simulink model "RPI_fuzzy"  (R2023b)
settings: Solver=ode3  StartTime=0.0  StopTime=inf  FixedStep=1  RelTol=1e-3  EnableMultiTasking=on
InitFcn:
  | rules_fuzzy_e_de=readfis('rules_fuzzy_e_de.fis');
values from neighbouring files (symbols this model uses):
  temp_ref = 22    [RPI_Fuzzy_script.m]    (also in plot_fuzzy.m = simout(:,1))
libraries: raspberrypiIOTlib x4, raspberrypiBasiclib x2, raspberrypienvironmentalsensorslib x1, fuzblock x1
settings Model: SimulationMode=external  ExtModeTrigDuration=2  Creator=marci  LastModifiedBy=marci
settings SolverCC: PositivePriorityOrder=on  AutoInsertRateTranBlk=on
settings OptimizationCC: EnhancedBackFolding=on  PassReuseOutputArgsAs=Individual arguments  ZeroExternalMemoryAtStartup=off  ZeroInternalMemoryAtStartup=off  MaxStackSize=64  OptimizeBlockOrder=speed  DifferentSizesBufferReuse=on  OptimizationCustomize=off  EfficientTunableParamExpr=on
settings DebuggingCC: ParameterTunabilityLossMsg=error
settings HardwareCC: ProdBitPerPointer=32  ProdBitPerSizeT=32  ProdBitPerPtrDiffT=32  ProdLargestAtomicInteger=Long  ProdLargestAtomicFloat=Double  ProdWordSize=32  ProdLongLongMode=on  ProdHWDeviceType=ARM Compatible->ARM Cortex
settings RTWCC: Description=Embedded Coder  SystemTargetFile=ert.tlc  HardwareBoard=Raspberry Pi  TemplateMakefile=ert_default_tmf  Toolchain=GNU GCC Embedded Linux  BuildConfiguration=Faster Runs
settings CodeAppCC: ForceParamTrailComments=on  IgnoreCustomStorageClasses=off  OperatorAnnotations=on  SimulinkDataObjDesc=on  SFDataObjDesc=on  InsertBlockDesc=on
settings ERTTargetCC: TargetLangStandard=C99 (ISO)  SupportContinuousTime=on  SupportVariableSizeSignals=on  ExtMode=on  ExtModeTransport=2  ExtModeStaticAlloc=on  ExtModeMaxTrigDuration=1000  ExtModeMexFile=ext_xcp  ExtModeMexArgs='192.168.0.236' 0 17725  ExtModeIntrfLevel=Level2 - Open

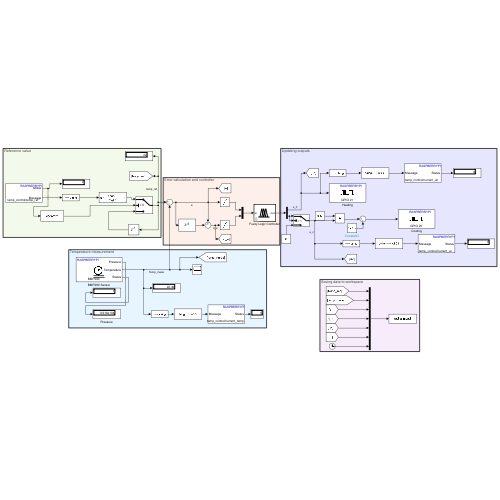
[thumbnail: Simulink's stored preview of the top-level diagram]
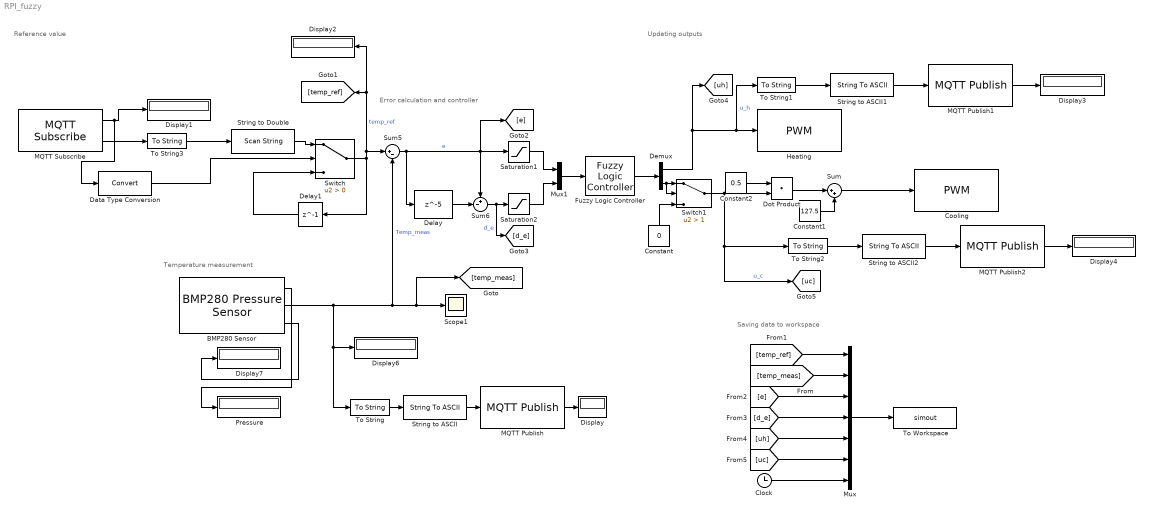
== system RPI_fuzzy ==
  note: Error calculation and controller
  note: Reference value
  note: Temperature measurement
  note: Saving data to workspace
  note: Updating outputs
  BMP280 Sensor : raspberrypienvironmentalsensorslib/BMP280 Pressure Sensor  I2CModule=1  I2CAddress=0x76  BitRate=1000000  IsActivePressure=on  IsActiveTemperature=on  IsStatus=on  FilterMode=0  PressureSensitivityFactor=2.62  TemperatureSensitivityFactor=0.005  DataType=double  SampleTime=1
  Clock : Clock
  Constant : Constant  Value=0
  Constant1 : Constant  Value=127.5
  Constant2 : Constant  Value=0.5
  Cooling : raspberrypiBasiclib/PWM  board=Pi 3 Model B  Pin_=20  Frequency=40  blockPlatform=Raspberry Pi
  Data Type Conversion : DataTypeConversion  SaturateOnIntegerOverflow=off  RndMeth=Floor
  Delay : Delay  DelayLength=5  InputProcessing=Columns as channels (frame based)  SampleTime=1
  Delay1 : Delay  DelayLength=1  InitialCondition=22
  Demux : Demux  Outputs=2
  Display{,1..4,6..7} (7 alike) : Display
  Dot Product : DotProduct  OutDataTypeStr=Inherit: Inherit via internal rule
  Fuzzy Logic Controller : fuzblock/Fuzzy Logic  Controller  FIS=rules_fuzzy_e_de  OutputSampleNumber=101  DataType=double  FuzzifiedInputs=off  RuleFiringStrengths=off  RuleOutputs=off  AggregatedOutputs=off  SimulateUsing=Interpreted execution  OutOfRangeInputValueMessage=warning  NoRuleFiredMessage=warning  EmptyOutputFuzzySetMessage=warning
  Heating : raspberrypiBasiclib/PWM  board=Pi 3 Model B  Pin_=21  Frequency=40  blockPlatform=Raspberry Pi
  MQTT Publish : raspberrypiIOTlib/MQTT Publish  Topic=temp_control/current_temp  QoS=0  RetainMsg=off  blockPlatform=RASPBERRYPI
  MQTT Publish1 : raspberrypiIOTlib/MQTT Publish  Topic=temp_control/current_uh  QoS=0  RetainMsg=off  blockPlatform=RASPBERRYPI
  MQTT Publish2 : raspberrypiIOTlib/MQTT Publish  Topic=temp_control/current_uc  QoS=0  RetainMsg=off  blockPlatform=RASPBERRYPI
  MQTT Subscribe : raspberrypiIOTlib/MQTT Subscribe  Topic=temp_control/temp_ref  QoS=0  MessageLength=1  OutputMessage=on  SampleTime=1  blockPlatform=RASPBERRYPI
  Mux : Mux  Inputs=7
  Mux1 : Mux  Inputs=2
  Pressure : Display
  Saturation1 : Saturate  UpperLimit=5  LowerLimit=-5
  Saturation2 : Saturate  UpperLimit=0.1  LowerLimit=-0.1
  Scope1 : Scope
  String to ASCII : StringToASCII
  String to ASCII1 : StringToASCII
  String to ASCII2 : StringToASCII
  String to Double : ScanString  Format="\"%lf\""
  Sum : Sum  Inputs=|++
  Sum5 : Sum  Inputs=|+-
  Sum6 : Sum  Inputs=+-|
  Switch : Switch  Criteria=u2 > Threshold  SaturateOnIntegerOverflow=off  InputSameDT=off
  Switch1 : Switch  Criteria=u2 > Threshold  Threshold=1  SaturateOnIntegerOverflow=off  InputSameDT=off
  To String{,1..3} (4 alike) : ToString
  To Workspace : ToWorkspace  VariableName=simout  SampleTime=1
  wires:
  Saturation1/1 -> Mux1/1
  BMP280 Sensor/2 -> Sum5/2, [temp_meas], Scope1/1, To String/1, Display6/1  "Temp_meas"
  Sum5/1 -> Delay/1, [e], Sum6/1, Saturation1/1  "e"
  Mux1/1 -> Fuzzy Logic Controller/1
  Saturation2/1 -> Mux1/2
  Sum6/1 -> [d_e], Saturation2/1  "d_e"
  Switch/1 -> Display2/1, [temp_ref], Sum5/1, Delay1/1  "temp_ref"
  Delay/1 -> Sum6/2
  BMP280 Sensor/3 -> Display7/1
  BMP280 Sensor/1 -> Pressure/1
  Fuzzy Logic Controller/1 -> Demux/1
  Demux/1 -> [uh], To String1/1, Heating/1  "u_h"
  Switch1/1 -> Dot Product/2, [uc], To String2/1  "u_c"
  [uc] -> Mux/6
  Clock/1 -> Mux/7
  [d_e] -> Mux/4
  [temp_ref] -> Mux/1
  [temp_meas] -> Mux/2
  Mux/1 -> To Workspace/1
  [uh] -> Mux/5
  [e] -> Mux/3
  MQTT Publish/1 -> Display/1
  To String/1 -> String to ASCII/1
  String to ASCII/1 -> MQTT Publish/1
  MQTT Subscribe/2 -> To String3/1
  String to Double/1 -> Switch/1
  To String1/1 -> String to ASCII1/1
  String to ASCII1/1 -> MQTT Publish1/1
  MQTT Publish1/1 -> Display3/1
  String to ASCII2/1 -> MQTT Publish2/1
  MQTT Publish2/1 -> Display4/1
  To String2/1 -> String to ASCII2/1
  MQTT Subscribe/1 -> Data Type Conversion/1, Display1/1
  Data Type Conversion/1 -> Switch/2
  To String3/1 -> String to Double/1
  Delay1/1 -> Switch/3
  Demux/2 -> Switch1/2, Switch1/1
  Constant/1 -> Switch1/3
  Dot Product/1 -> Sum/1
  Sum/1 -> Cooling/1
  Constant1/1 -> Sum/2
  Constant2/1 -> Dot Product/1
